simulink model "Chua"  (R2014b)
settings: Solver=ode45  StartTime=0.0  StopTime=10.0  RelTol=1e-3
values from neighbouring files (symbols this model uses):
  a = 0.95    [Run_Aizawa.m]    (also in Run_Arneodo.m = -5.5; Run_Chen.m = 33; Run_Chua.m = 15.6; Run_Chua_4D.m = 0.03)
  b = 0.7    [Run_Aizawa.m]    (also in Run_Arneodo.m = 3.5; Run_Chen.m = 3; Run_Chua.m = 28; Run_Duffing.m = 100)
  m0 = -1.143    [Run_Chua.m]
  m1 = -0.714    [Run_Chua.m]
undefined symbols (not defined in the file or in its folder): param
settings Model: Creator=Arek  LastModifiedBy=Arek

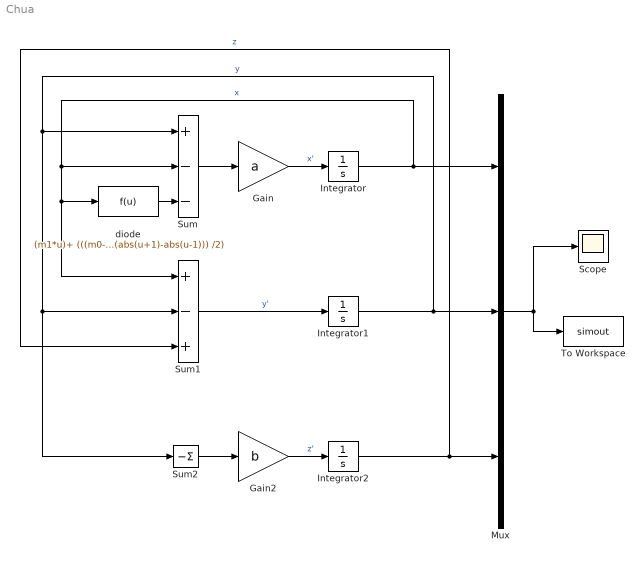
== system Chua ==
  Gain : Gain  Gain=a
  Gain2 : Gain  Gain=b
  Integrator : Integrator  InitialCondition=param.ic(1)
  Integrator1 : Integrator  InitialCondition=param.ic(2)
  Integrator2 : Integrator  InitialCondition=param.ic(3)
  Mux : Mux  Inputs=3
  Scope : Scope
      settings: ShowLegends=on  TimeRange=0.05  YMin=-6  YMax=2
  Sum : Sum  Inputs=+--
  Sum1 : Sum  Inputs=+-+
  Sum2 : Sum  Inputs=-
  To Workspace : ToWorkspace  VariableName=simout  SaveFormat=Timeseries  SampleTime=-1
  diode : Fcn  Expr=(m1*u)+ (((m0-m1) * (abs(u+1)-abs(u-1))) /2)
  wires:
  Gain2/1 -> Integrator2/1  "z'"
  Sum1/1 -> Integrator1/1  "y'"
  Gain/1 -> Integrator/1  "x'"
  Sum/1 -> Gain/1
  Integrator/1 -> Sum1/1, diode/1, Sum/2, Mux/1  "x"
  Integrator1/1 -> Sum/1, Sum2/1, Sum1/2, Mux/2  "y"
  Integrator2/1 -> Sum1/3, Mux/3  "z"
  Mux/1 -> Scope/1, To Workspace/1
  Sum2/1 -> Gain2/1
  diode/1 -> Sum/3
